simulink model "drone"  (R2020b)
settings: Solver=VariableStepAuto  StartTime=0.0  StopTime=3  RelTol=1e-3
values from neighbouring files (symbols this model uses):
  planta = obterPlanta()    [simularDrone.m]
  proj = obterProjeto()    [simularDrone.m]
libraries: pid_lib x6
settings Model: EnablePacing=on  Creator=kowalks  LastModifiedBy=kenji

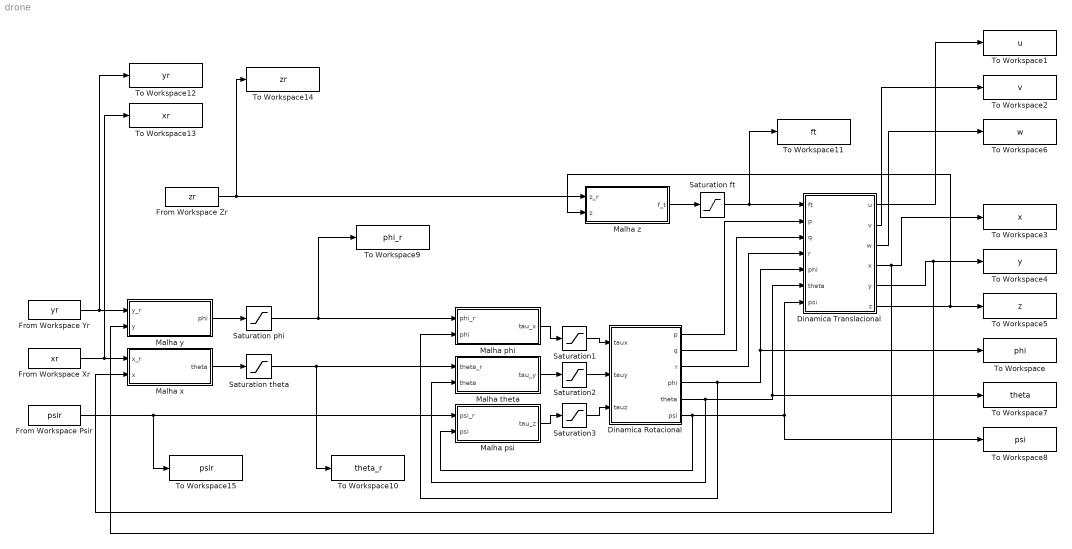
== system drone ==
  Dinamica Rotacional : Subsystem
  Dinamica Translacional : Subsystem
  From Workspace Psir : FromWorkspace  VariableName=psir
  From Workspace Xr : FromWorkspace  VariableName=xr
  From Workspace Yr : FromWorkspace  VariableName=yr
  From Workspace Zr : FromWorkspace  VariableName=zr
  Malha phi : Subsystem
  Malha psi : Subsystem
  Malha theta : Subsystem
  Malha x : Subsystem
  Malha y : Subsystem
  Malha z : Subsystem
  Saturation ft : Saturate  UpperLimit=2*planta.m*planta.g  LowerLimit=0.1*planta.m*planta.g
  Saturation phi : Saturate  UpperLimit=pi/6  LowerLimit=-pi/6
  Saturation theta : Saturate  UpperLimit=pi/6  LowerLimit=-pi/6
  Saturation1 : Saturate  UpperLimit=2*sqrt(2)*planta.l*planta.m*planta.g  LowerLimit=-2*sqrt(2)*planta.l*planta.m*planta.g
  Saturation2 : Saturate  UpperLimit=2*sqrt(2)*planta.l*planta.m*planta.g  LowerLimit=-2*sqrt(2)*planta.l*planta.m*planta.g
  Saturation3 : Saturate  UpperLimit=2*sqrt(2)*planta.l*planta.m*planta.g  LowerLimit=-2*sqrt(2)*planta.l*planta.m*planta.g
  To Workspace : ToWorkspace  VariableName=phi  SaveFormat=Timeseries  SampleTime=-1
  To Workspace1 : ToWorkspace  VariableName=u  SaveFormat=Timeseries  SampleTime=-1
  To Workspace10 : ToWorkspace  VariableName=theta_r  SaveFormat=Timeseries  SampleTime=-1
  To Workspace11 : ToWorkspace  VariableName=ft  SaveFormat=Timeseries  SampleTime=-1
  To Workspace12 : ToWorkspace  VariableName=yr  SaveFormat=Timeseries  SampleTime=-1
  To Workspace13 : ToWorkspace  VariableName=xr  SaveFormat=Timeseries  SampleTime=-1
  To Workspace14 : ToWorkspace  VariableName=zr  SaveFormat=Timeseries  SampleTime=-1
  To Workspace15 : ToWorkspace  VariableName=psir  SaveFormat=Timeseries  SampleTime=-1
  To Workspace2 : ToWorkspace  VariableName=v  SaveFormat=Timeseries  SampleTime=-1
  To Workspace3 : ToWorkspace  VariableName=x  SaveFormat=Timeseries  SampleTime=-1
  To Workspace4 : ToWorkspace  VariableName=y  SaveFormat=Timeseries  SampleTime=-1
  To Workspace5 : ToWorkspace  VariableName=z  SaveFormat=Timeseries  SampleTime=-1
  To Workspace6 : ToWorkspace  VariableName=w  SaveFormat=Timeseries  SampleTime=-1
  To Workspace7 : ToWorkspace  VariableName=theta  SaveFormat=Timeseries  SampleTime=-1
  To Workspace8 : ToWorkspace  VariableName=psi  SaveFormat=Timeseries  SampleTime=-1
  To Workspace9 : ToWorkspace  VariableName=phi_r  SaveFormat=Timeseries  SampleTime=-1
  wires:
  Dinamica Rotacional/6(psi) -> Malha psi/2(psi), Dinamica Translacional/7(psi), To Workspace8/1
  Dinamica Rotacional/5(theta) -> Malha theta/2(theta), To Workspace7/1, Dinamica Translacional/6(theta)
  Dinamica Rotacional/3(r) -> Dinamica Translacional/4(r)
  Dinamica Rotacional/2(q) -> Dinamica Translacional/3(q)
  Dinamica Rotacional/1(p) -> Dinamica Translacional/2(p)
  Dinamica Translacional/6(z) -> Malha z/2(z), To Workspace5/1
  Dinamica Translacional/5(y) -> Malha y/2(y), To Workspace4/1
  Dinamica Translacional/4(x) -> Malha x/2(x), To Workspace3/1
  Dinamica Translacional/3(w) -> To Workspace6/1
  Dinamica Translacional/2(v) -> To Workspace2/1
  Dinamica Translacional/1(u) -> To Workspace1/1
  From Workspace Xr/1 -> To Workspace13/1, Malha x/1(x_r)
  From Workspace Yr/1 -> To Workspace12/1, Malha y/1(y_r)
  From Workspace Psir/1 -> To Workspace15/1, Malha psi/1(psi_r)
  From Workspace Zr/1 -> To Workspace14/1, Malha z/1(z_r)
  Dinamica Rotacional/4(phi) -> Malha phi/2(phi), Dinamica Translacional/5(phi), To Workspace/1
  Malha y/1(phi) -> Saturation phi/1
  Malha x/1(theta) -> Saturation theta/1
  Saturation phi/1 -> To Workspace9/1, Malha phi/1(phi_r)
  Saturation theta/1 -> To Workspace10/1, Malha theta/1(theta_r)
  Malha z/1(f_t) -> Saturation ft/1
  Saturation ft/1 -> To Workspace11/1, Dinamica Translacional/1(ft)
  Malha phi/1(tau_x) -> Saturation1/1
  Saturation1/1 -> Dinamica Rotacional/1(taux)
  Saturation2/1 -> Dinamica Rotacional/2(tauy)
  Malha theta/1(tau_y) -> Saturation2/1
  Malha psi/1(tau_z) -> Saturation3/1
  Saturation3/1 -> Dinamica Rotacional/3(tauz)

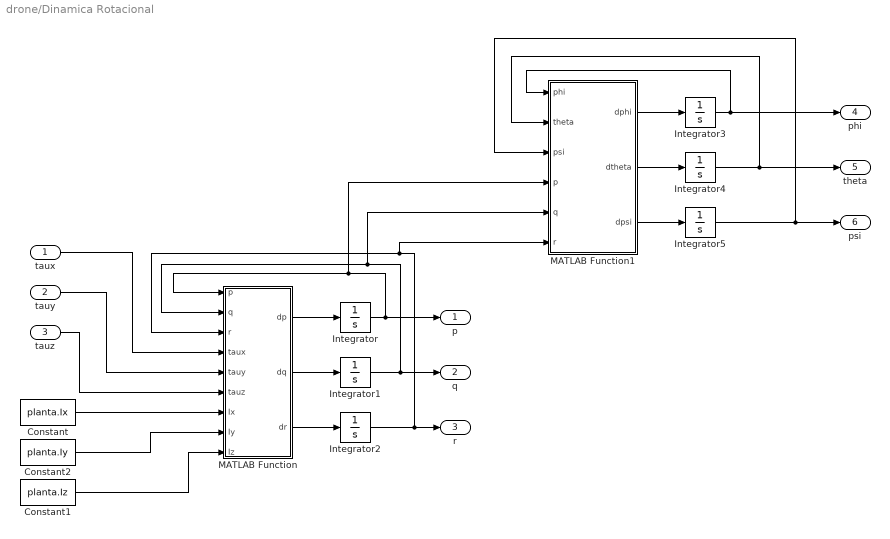
== system drone/Dinamica Rotacional ==
  taux : Inport
  tauy : Inport  Port=2
  tauz : Inport  Port=3
  Constant : Constant  Value=planta.Ix
  Constant1 : Constant  Value=planta.Iz
  Constant2 : Constant  Value=planta.Iy
  Integrator{,1..5} (6 alike) : Integrator
  MATLAB Function : MATLAB Function  TreatAsAtomicUnit=on
  MATLAB Function1 : MATLAB Function  TreatAsAtomicUnit=on
  p : Outport
  q : Outport  Port=2
  r : Outport  Port=3
  phi : Outport  Port=4
  theta : Outport  Port=5
  psi : Outport  Port=6
  wires:
  taux/1 -> MATLAB Function/4(taux)
  tauy/1 -> MATLAB Function/5(tauy)
  tauz/1 -> MATLAB Function/6(tauz)
  MATLAB Function/1(dp) -> Integrator/1
  MATLAB Function/2(dq) -> Integrator1/1
  MATLAB Function/3(dr) -> Integrator2/1
  Integrator1/1 -> q/1, MATLAB Function1/5(q), MATLAB Function/2(q)
  Integrator2/1 -> r/1, MATLAB Function1/6(r), MATLAB Function/3(r)
  Integrator/1 -> p/1, MATLAB Function1/4(p), MATLAB Function/1(p)
  Constant/1 -> MATLAB Function/7(Ix)
  Constant2/1 -> MATLAB Function/8(Iy)
  Constant1/1 -> MATLAB Function/9(Iz)
  MATLAB Function1/1(dphi) -> Integrator3/1
  MATLAB Function1/2(dtheta) -> Integrator4/1
  MATLAB Function1/3(dpsi) -> Integrator5/1
  Integrator3/1 -> MATLAB Function1/1(phi), phi/1
  Integrator4/1 -> theta/1, MATLAB Function1/2(theta)
  Integrator5/1 -> MATLAB Function1/3(psi), psi/1

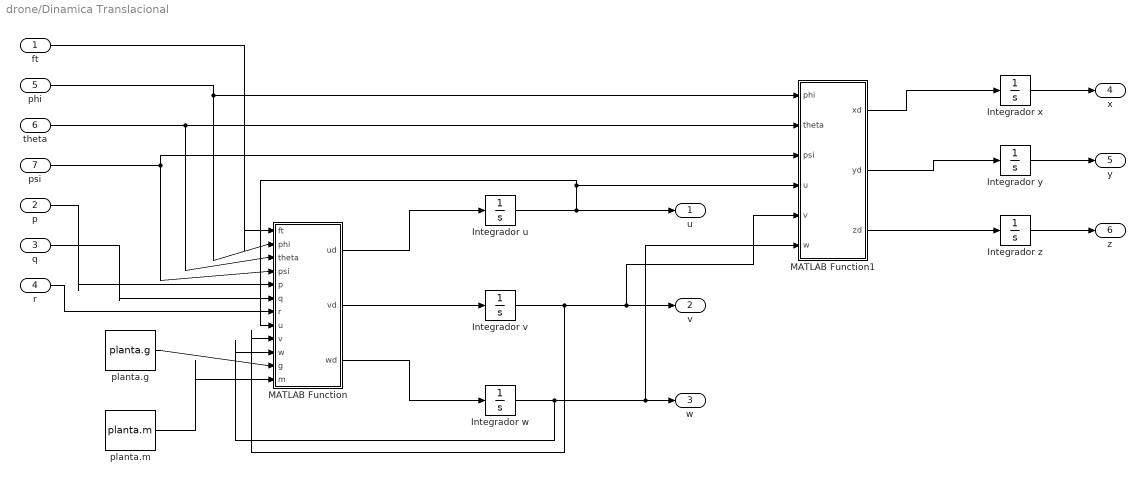
== system drone/Dinamica Translacional ==
  ft : Inport
  p : Inport  Port=2
  q : Inport  Port=3
  r : Inport  Port=4
  phi : Inport  Port=5
  theta : Inport  Port=6
  psi : Inport  Port=7
  Integrador u : Integrator
  Integrador v : Integrator
  Integrador w : Integrator
  Integrador x : Integrator
  Integrador y : Integrator
  Integrador z : Integrator
  MATLAB Function : MATLAB Function  TreatAsAtomicUnit=on
  MATLAB Function1 : MATLAB Function  TreatAsAtomicUnit=on
  planta.g : Constant  Value=planta.g
  planta.m : Constant  Value=planta.m
  u : Outport  PortDimensions=1
  v : Outport  Port=2  PortDimensions=1
  w : Outport  Port=3  PortDimensions=1
  x : Outport  Port=4  PortDimensions=1
  y : Outport  Port=5  PortDimensions=1
  z : Outport  Port=6  PortDimensions=1
  wires:
  phi/1 -> MATLAB Function/2(phi), MATLAB Function1/1(phi)
  theta/1 -> MATLAB Function/3(theta), MATLAB Function1/2(theta)
  psi/1 -> MATLAB Function/4(psi), MATLAB Function1/3(psi)
  ft/1 -> MATLAB Function/1(ft)
  MATLAB Function/1(ud) -> Integrador u/1
  MATLAB Function/2(vd) -> Integrador v/1
  MATLAB Function/3(wd) -> Integrador w/1
  Integrador w/1 -> MATLAB Function1/6(w), w/1, MATLAB Function/10(w)
  Integrador u/1 -> MATLAB Function/8(u), MATLAB Function1/4(u), u/1
  MATLAB Function1/2(yd) -> Integrador y/1
  MATLAB Function1/1(xd) -> Integrador x/1
  MATLAB Function1/3(zd) -> Integrador z/1
  p/1 -> MATLAB Function/5(p)
  q/1 -> MATLAB Function/6(q)
  r/1 -> MATLAB Function/7(r)
  Integrador v/1 -> MATLAB Function1/5(v), v/1, MATLAB Function/9(v)
  Integrador x/1 -> x/1
  Integrador y/1 -> y/1
  Integrador z/1 -> z/1
  planta.g/1 -> MATLAB Function/11(g)
  planta.m/1 -> MATLAB Function/12(m)

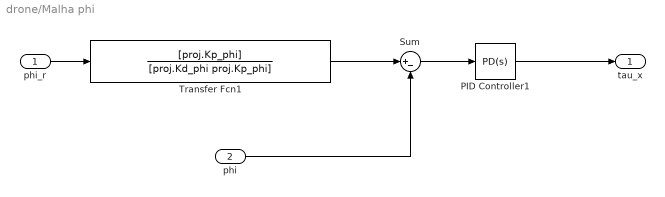
== system drone/Malha phi ==
  phi_r : Inport
  phi : Inport  Port=2
  PID Controller1 : pid_lib/PID Controller  Controller=PD  Form=Parallel  TimeDomain=Continuous-time  UseExternalTs=off  SampleTime=-1  IntegratorMethod=Forward Euler  FilterMethod=Forward Euler  ControllerParametersSource=internal  P=proj.Kp_phi  I=1  D=proj.Kd_phi  UseFilter=on  N=10000  TunerSelectOption=Transfer Function Based (PID Tuner App)  InitialConditionSource=internal  InitialConditionForIntegrator=0  InitialConditionForFilter=0  DifferentiatorICPrevScaledInput=0  ExternalReset=none  TrackingMode=off  Kt=1  LimitOutput=off  SatLimitsSource=internal  UpperSaturationLimit=inf  LowerSaturationLimit=-inf  LinearizeAsGain=on  AntiWindupMode=none  Kb=1  POutMin=[]  POutMax=[]  IOutMin=[]  IOutMax=[]  DOutMin=[]  DOutMax=[]  NOutMin=[]  NOutMax=[]  SumOutMin=[]  SumOutMax=[]  SaturationOutMin=[]  SaturationOutMax=[]  PParamMin=[]  PParamMax=[]  IParamMin=[]  IParamMax=[]  DParamMin=[]  DParamMax=[]  NParamMin=[]  NParamMax=[]  KbParamMin=[]  KbParamMax=[]  KtParamMin=[]  KtParamMax=[]  KbOutMin=[]  KbOutMax=[]  KtOutMin=[]  KtOutMax=[]  IntegratorOutMin=[]  IntegratorOutMax=[]  FilterOutMin=[]  FilterOutMax=[]  SumI1OutMin=[]  SumI1OutMax=[]  SumI2OutMin=[]  SumI2OutMax=[]  SumI3OutMin=[]  SumI3OutMax=[]  SumI4OutMin=[]  SumI4OutMax=[]  SumDOutMin=[]  SumDOutMax=[]  DifferentiatorOutMin=[]  DifferentiatorOutMax=[]  FilterDiffOutCoefMin=[]  FilterDiffOutCoefMax=[]  ReciprocalOutMin=[]  ReciprocalOutMax=[]  SumDenOutMin=[]  SumDenOutMax=[]  SumNumOutMin=[]  SumNumOutMax=[]  DivideOutMin=[]  DivideOutMax=[]  UdiffTsProdOutMin=[]  UdiffTsProdOutMax=[]  NTsProdOutMin=[]  NTsProdOutMax=[]  UintegralTsProdOutMin=[]  UintegralTsProdOutMax=[]  UngainTsProdOutMin=[]  UngainTsProdOutMax=[]  IntegratorContinuousStateAttributes=''  IntegratorStateMustResolveToSignalObject=off  IntegratorRTWStateStorageClass=Auto  FilterContinuousStateAttributes=''  FilterStateMustResolveToSignalObject=off  FilterRTWStateStorageClass=Auto  ParallelPVariant=InternalParameters  IdealPVariant=Disabled  IVariant=Disabled  DVariant=InternalParameters  IntegratorVariant=Disabled  SatVariant=Disabled  AWVariant=Disabled  PCopyVariant=Disabled  TRVariant=Disabled  FdbkBlocksVariant=Forward  IdealPFdbkVariant=Disabled  SatFdbkVariant=Disabled  DerivativeFilterVariant=ContFilter  NVariant=InternalParameters  NCopyVariant=Disabled  FilterICVariant=InternalICsFilter  IntegratorICVariant=Disabled  ExternalResetVariant=Disabled  TRSumVariant=Passthrough  SumFdbkVariant=Disabled  SumVariant=Sum_PD  TsampFilterVariant=InternalTs  TsampNgainVariant=Passthrough  TsampIntegralVariant=Disabled_SignalSpec  ExternalSaturationOutDataTypeStr=Inherit: Same as second input
  Sum : Sum  Inputs=|+-
  Transfer Fcn1 : TransferFcn  Numerator=[proj.Kp_phi]  Denominator=[proj.Kd_phi proj.Kp_phi]
  tau_x : Outport
  wires:
  phi_r/1 -> Transfer Fcn1/1
  Sum/1 -> PID Controller1/1
  Transfer Fcn1/1 -> Sum/1
  PID Controller1/1 -> tau_x/1
  phi/1 -> Sum/2

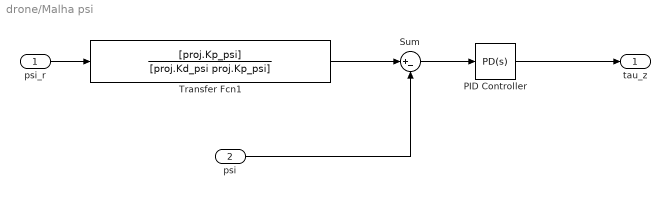
== system drone/Malha psi ==
  psi_r : Inport
  psi : Inport  Port=2
  PID Controller : pid_lib/PID Controller  Controller=PD  Form=Parallel  TimeDomain=Continuous-time  UseExternalTs=off  SampleTime=-1  IntegratorMethod=Forward Euler  FilterMethod=Forward Euler  ControllerParametersSource=internal  P=proj.Kp_psi  I=1  D=proj.Kd_psi  UseFilter=on  N=10000  TunerSelectOption=Transfer Function Based (PID Tuner App)  InitialConditionSource=internal  InitialConditionForIntegrator=0  InitialConditionForFilter=0  DifferentiatorICPrevScaledInput=0  ExternalReset=none  TrackingMode=off  Kt=1  LimitOutput=off  SatLimitsSource=internal  UpperSaturationLimit=inf  LowerSaturationLimit=-inf  LinearizeAsGain=on  AntiWindupMode=none  Kb=1  POutMin=[]  POutMax=[]  IOutMin=[]  IOutMax=[]  DOutMin=[]  DOutMax=[]  NOutMin=[]  NOutMax=[]  SumOutMin=[]  SumOutMax=[]  SaturationOutMin=[]  SaturationOutMax=[]  PParamMin=[]  PParamMax=[]  IParamMin=[]  IParamMax=[]  DParamMin=[]  DParamMax=[]  NParamMin=[]  NParamMax=[]  KbParamMin=[]  KbParamMax=[]  KtParamMin=[]  KtParamMax=[]  KbOutMin=[]  KbOutMax=[]  KtOutMin=[]  KtOutMax=[]  IntegratorOutMin=[]  IntegratorOutMax=[]  FilterOutMin=[]  FilterOutMax=[]  SumI1OutMin=[]  SumI1OutMax=[]  SumI2OutMin=[]  SumI2OutMax=[]  SumI3OutMin=[]  SumI3OutMax=[]  SumI4OutMin=[]  SumI4OutMax=[]  SumDOutMin=[]  SumDOutMax=[]  DifferentiatorOutMin=[]  DifferentiatorOutMax=[]  FilterDiffOutCoefMin=[]  FilterDiffOutCoefMax=[]  ReciprocalOutMin=[]  ReciprocalOutMax=[]  SumDenOutMin=[]  SumDenOutMax=[]  SumNumOutMin=[]  SumNumOutMax=[]  DivideOutMin=[]  DivideOutMax=[]  UdiffTsProdOutMin=[]  UdiffTsProdOutMax=[]  NTsProdOutMin=[]  NTsProdOutMax=[]  UintegralTsProdOutMin=[]  UintegralTsProdOutMax=[]  UngainTsProdOutMin=[]  UngainTsProdOutMax=[]  IntegratorContinuousStateAttributes=''  IntegratorStateMustResolveToSignalObject=off  IntegratorRTWStateStorageClass=Auto  FilterContinuousStateAttributes=''  FilterStateMustResolveToSignalObject=off  FilterRTWStateStorageClass=Auto  ParallelPVariant=InternalParameters  IdealPVariant=Disabled  IVariant=Disabled  DVariant=InternalParameters  IntegratorVariant=Disabled  SatVariant=Disabled  AWVariant=Disabled  PCopyVariant=Disabled  TRVariant=Disabled  FdbkBlocksVariant=Forward  IdealPFdbkVariant=Disabled  SatFdbkVariant=Disabled  DerivativeFilterVariant=ContFilter  NVariant=InternalParameters  NCopyVariant=Disabled  FilterICVariant=InternalICsFilter  IntegratorICVariant=Disabled  ExternalResetVariant=Disabled  TRSumVariant=Passthrough  SumFdbkVariant=Disabled  SumVariant=Sum_PD  TsampFilterVariant=InternalTs  TsampNgainVariant=Passthrough  TsampIntegralVariant=Disabled_SignalSpec  ExternalSaturationOutDataTypeStr=Inherit: Same as second input
  Sum : Sum  Inputs=|+-
  Transfer Fcn1 : TransferFcn  Numerator=[proj.Kp_psi]  Denominator=[proj.Kd_psi proj.Kp_psi]
  tau_z : Outport
  wires:
  psi/1 -> Sum/2
  PID Controller/1 -> tau_z/1
  psi_r/1 -> Transfer Fcn1/1
  Transfer Fcn1/1 -> Sum/1
  Sum/1 -> PID Controller/1

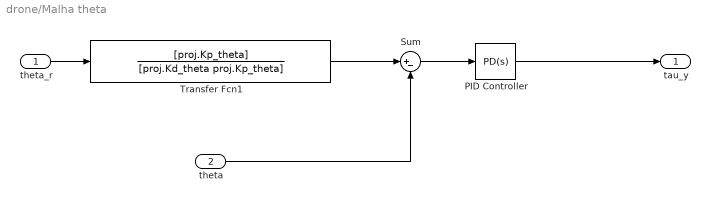
== system drone/Malha theta ==
  theta_r : Inport
  theta : Inport  Port=2
  PID Controller : pid_lib/PID Controller  Controller=PD  Form=Parallel  TimeDomain=Continuous-time  UseExternalTs=off  SampleTime=-1  IntegratorMethod=Forward Euler  FilterMethod=Forward Euler  ControllerParametersSource=internal  P=proj.Kp_theta  I=1  D=proj.Kd_theta  UseFilter=on  N=10000  TunerSelectOption=Transfer Function Based (PID Tuner App)  InitialConditionSource=internal  InitialConditionForIntegrator=0  InitialConditionForFilter=0  DifferentiatorICPrevScaledInput=0  ExternalReset=none  TrackingMode=off  Kt=1  LimitOutput=off  SatLimitsSource=internal  UpperSaturationLimit=planta.g*pi/6  LowerSaturationLimit=-planta.g*pi/6  LinearizeAsGain=off  AntiWindupMode=back-calculation  Kb=1  POutMin=[]  POutMax=[]  IOutMin=[]  IOutMax=[]  DOutMin=[]  DOutMax=[]  NOutMin=[]  NOutMax=[]  SumOutMin=[]  SumOutMax=[]  SaturationOutMin=[]  SaturationOutMax=[]  PParamMin=[]  PParamMax=[]  IParamMin=[]  IParamMax=[]  DParamMin=[]  DParamMax=[]  NParamMin=[]  NParamMax=[]  KbParamMin=[]  KbParamMax=[]  KtParamMin=[]  KtParamMax=[]  KbOutMin=[]  KbOutMax=[]  KtOutMin=[]  KtOutMax=[]  IntegratorOutMin=[]  IntegratorOutMax=[]  FilterOutMin=[]  FilterOutMax=[]  SumI1OutMin=[]  SumI1OutMax=[]  SumI2OutMin=[]  SumI2OutMax=[]  SumI3OutMin=[]  SumI3OutMax=[]  SumI4OutMin=[]  SumI4OutMax=[]  SumDOutMin=[]  SumDOutMax=[]  DifferentiatorOutMin=[]  DifferentiatorOutMax=[]  FilterDiffOutCoefMin=[]  FilterDiffOutCoefMax=[]  ReciprocalOutMin=[]  ReciprocalOutMax=[]  SumDenOutMin=[]  SumDenOutMax=[]  SumNumOutMin=[]  SumNumOutMax=[]  DivideOutMin=[]  DivideOutMax=[]  UdiffTsProdOutMin=[]  UdiffTsProdOutMax=[]  NTsProdOutMin=[]  NTsProdOutMax=[]  UintegralTsProdOutMin=[]  UintegralTsProdOutMax=[]  UngainTsProdOutMin=[]  UngainTsProdOutMax=[]  IntegratorContinuousStateAttributes=''  IntegratorStateMustResolveToSignalObject=off  IntegratorRTWStateStorageClass=Auto  FilterContinuousStateAttributes=''  FilterStateMustResolveToSignalObject=off  FilterRTWStateStorageClass=Auto  ParallelPVariant=InternalParameters  IdealPVariant=Disabled  IVariant=Disabled  DVariant=InternalParameters  IntegratorVariant=Disabled  SatVariant=Disabled  AWVariant=Disabled  PCopyVariant=Disabled  TRVariant=Disabled  FdbkBlocksVariant=Forward  IdealPFdbkVariant=Disabled  SatFdbkVariant=Disabled  DerivativeFilterVariant=ContFilter  NVariant=InternalParameters  NCopyVariant=Disabled  FilterICVariant=InternalICsFilter  IntegratorICVariant=Disabled  ExternalResetVariant=Disabled  TRSumVariant=Passthrough  SumFdbkVariant=Disabled  SumVariant=Sum_PD  TsampFilterVariant=InternalTs  TsampNgainVariant=Passthrough  TsampIntegralVariant=Disabled_SignalSpec  ExternalSaturationOutDataTypeStr=Inherit: Same as second input
  Sum : Sum  Inputs=|+-
  Transfer Fcn1 : TransferFcn  Numerator=[proj.Kp_theta]  Denominator=[proj.Kd_theta proj.Kp_theta]
  tau_y : Outport
  wires:
  theta_r/1 -> Transfer Fcn1/1
  Sum/1 -> PID Controller/1
  Transfer Fcn1/1 -> Sum/1
  theta/1 -> Sum/2
  PID Controller/1 -> tau_y/1

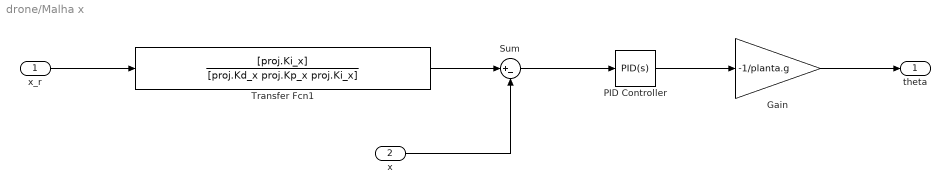
== system drone/Malha x ==
  x_r : Inport
  x : Inport  Port=2
  Gain : Gain  Gain=-1/planta.g
  PID Controller : pid_lib/PID Controller  Controller=PID  Form=Parallel  TimeDomain=Continuous-time  UseExternalTs=off  SampleTime=-1  IntegratorMethod=Forward Euler  FilterMethod=Forward Euler  ControllerParametersSource=internal  P=proj.Kp_x  I=proj.Ki_x  D=proj.Kd_x  UseFilter=on  N=10000000  TunerSelectOption=Transfer Function Based (PID Tuner App)  InitialConditionSource=internal  InitialConditionForIntegrator=0  InitialConditionForFilter=0  DifferentiatorICPrevScaledInput=0  ExternalReset=none  TrackingMode=off  Kt=1  LimitOutput=on  SatLimitsSource=internal  UpperSaturationLimit=planta.g*pi/6  LowerSaturationLimit=-planta.g*pi/6  LinearizeAsGain=off  AntiWindupMode=back-calculation  Kb=8  POutMin=[]  POutMax=[]  IOutMin=[]  IOutMax=[]  DOutMin=[]  DOutMax=[]  NOutMin=[]  NOutMax=[]  SumOutMin=[]  SumOutMax=[]  SaturationOutMin=[]  SaturationOutMax=[]  PParamMin=[]  PParamMax=[]  IParamMin=[]  IParamMax=[]  DParamMin=[]  DParamMax=[]  NParamMin=[]  NParamMax=[]  KbParamMin=[]  KbParamMax=[]  KtParamMin=[]  KtParamMax=[]  KbOutMin=[]  KbOutMax=[]  KtOutMin=[]  KtOutMax=[]  IntegratorOutMin=[]  IntegratorOutMax=[]  FilterOutMin=[]  FilterOutMax=[]  SumI1OutMin=[]  SumI1OutMax=[]  SumI2OutMin=[]  SumI2OutMax=[]  SumI3OutMin=[]  SumI3OutMax=[]  SumI4OutMin=[]  SumI4OutMax=[]  SumDOutMin=[]  SumDOutMax=[]  DifferentiatorOutMin=[]  DifferentiatorOutMax=[]  FilterDiffOutCoefMin=[]  FilterDiffOutCoefMax=[]  ReciprocalOutMin=[]  ReciprocalOutMax=[]  SumDenOutMin=[]  SumDenOutMax=[]  SumNumOutMin=[]  SumNumOutMax=[]  DivideOutMin=[]  DivideOutMax=[]  UdiffTsProdOutMin=[]  UdiffTsProdOutMax=[]  NTsProdOutMin=[]  NTsProdOutMax=[]  UintegralTsProdOutMin=[]  UintegralTsProdOutMax=[]  UngainTsProdOutMin=[]  UngainTsProdOutMax=[]  IntegratorContinuousStateAttributes=''  IntegratorStateMustResolveToSignalObject=off  IntegratorRTWStateStorageClass=Auto  FilterContinuousStateAttributes=''  FilterStateMustResolveToSignalObject=off  FilterRTWStateStorageClass=Auto  ParallelPVariant=InternalParameters  IdealPVariant=Disabled  IVariant=InternalParameters  DVariant=InternalParameters  IntegratorVariant=Continuous  SatVariant=Enabled  AWVariant=BackCalculation  PCopyVariant=Disabled  TRVariant=Disabled  FdbkBlocksVariant=Forward  IdealPFdbkVariant=Disabled  SatFdbkVariant=Disabled  DerivativeFilterVariant=ContFilter  NVariant=InternalParameters  NCopyVariant=Disabled  FilterICVariant=InternalICsFilter  IntegratorICVariant=InternalICs  ExternalResetVariant=Disabled  TRSumVariant=Passthrough  SumFdbkVariant=Disabled  SumVariant=Sum_PID  TsampFilterVariant=InternalTs  TsampNgainVariant=Passthrough  TsampIntegralVariant=Passthrough  ExternalSaturationOutDataTypeStr=Inherit: Same as second input
  Sum : Sum  Inputs=|+-
  Transfer Fcn1 : TransferFcn  Numerator=[proj.Ki_x]  Denominator=[proj.Kd_x proj.Kp_x proj.Ki_x]
  theta : Outport
  wires:
  Transfer Fcn1/1 -> Sum/1
  x/1 -> Sum/2
  x_r/1 -> Transfer Fcn1/1
  Sum/1 -> PID Controller/1
  PID Controller/1 -> Gain/1
  Gain/1 -> theta/1

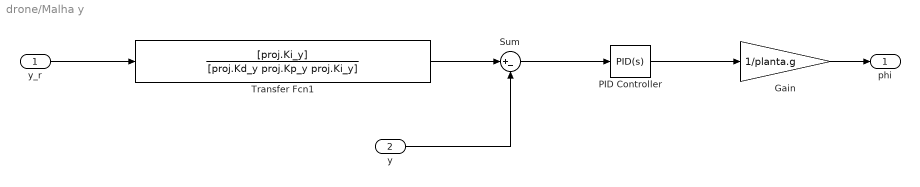
== system drone/Malha y ==
  y_r : Inport
  y : Inport  Port=2
  Gain : Gain  Gain=1/planta.g
  PID Controller : pid_lib/PID Controller  Controller=PID  Form=Parallel  TimeDomain=Continuous-time  UseExternalTs=off  SampleTime=-1  IntegratorMethod=Forward Euler  FilterMethod=Forward Euler  ControllerParametersSource=internal  P=proj.Kp_y  I=proj.Ki_y  D=proj.Kd_y  UseFilter=on  N=10000000  TunerSelectOption=Transfer Function Based (PID Tuner App)  InitialConditionSource=internal  InitialConditionForIntegrator=0  InitialConditionForFilter=0  DifferentiatorICPrevScaledInput=0  ExternalReset=none  TrackingMode=off  Kt=1  LimitOutput=on  SatLimitsSource=internal  UpperSaturationLimit=planta.g*pi/6  LowerSaturationLimit=-planta.g*pi/6  LinearizeAsGain=off  AntiWindupMode=back-calculation  Kb=8  POutMin=[]  POutMax=[]  IOutMin=[]  IOutMax=[]  DOutMin=[]  DOutMax=[]  NOutMin=[]  NOutMax=[]  SumOutMin=[]  SumOutMax=[]  SaturationOutMin=[]  SaturationOutMax=[]  PParamMin=[]  PParamMax=[]  IParamMin=[]  IParamMax=[]  DParamMin=[]  DParamMax=[]  NParamMin=[]  NParamMax=[]  KbParamMin=[]  KbParamMax=[]  KtParamMin=[]  KtParamMax=[]  KbOutMin=[]  KbOutMax=[]  KtOutMin=[]  KtOutMax=[]  IntegratorOutMin=[]  IntegratorOutMax=[]  FilterOutMin=[]  FilterOutMax=[]  SumI1OutMin=[]  SumI1OutMax=[]  SumI2OutMin=[]  SumI2OutMax=[]  SumI3OutMin=[]  SumI3OutMax=[]  SumI4OutMin=[]  SumI4OutMax=[]  SumDOutMin=[]  SumDOutMax=[]  DifferentiatorOutMin=[]  DifferentiatorOutMax=[]  FilterDiffOutCoefMin=[]  FilterDiffOutCoefMax=[]  ReciprocalOutMin=[]  ReciprocalOutMax=[]  SumDenOutMin=[]  SumDenOutMax=[]  SumNumOutMin=[]  SumNumOutMax=[]  DivideOutMin=[]  DivideOutMax=[]  UdiffTsProdOutMin=[]  UdiffTsProdOutMax=[]  NTsProdOutMin=[]  NTsProdOutMax=[]  UintegralTsProdOutMin=[]  UintegralTsProdOutMax=[]  UngainTsProdOutMin=[]  UngainTsProdOutMax=[]  IntegratorContinuousStateAttributes=''  IntegratorStateMustResolveToSignalObject=off  IntegratorRTWStateStorageClass=Auto  FilterContinuousStateAttributes=''  FilterStateMustResolveToSignalObject=off  FilterRTWStateStorageClass=Auto  ParallelPVariant=InternalParameters  IdealPVariant=Disabled  IVariant=InternalParameters  DVariant=InternalParameters  IntegratorVariant=Continuous  SatVariant=Enabled  AWVariant=BackCalculation  PCopyVariant=Disabled  TRVariant=Disabled  FdbkBlocksVariant=Forward  IdealPFdbkVariant=Disabled  SatFdbkVariant=Disabled  DerivativeFilterVariant=ContFilter  NVariant=InternalParameters  NCopyVariant=Disabled  FilterICVariant=InternalICsFilter  IntegratorICVariant=InternalICs  ExternalResetVariant=Disabled  TRSumVariant=Passthrough  SumFdbkVariant=Disabled  SumVariant=Sum_PID  TsampFilterVariant=InternalTs  TsampNgainVariant=Passthrough  TsampIntegralVariant=Passthrough  ExternalSaturationOutDataTypeStr=Inherit: Same as second input
  Sum : Sum  Inputs=|+-
  Transfer Fcn1 : TransferFcn  Numerator=[proj.Ki_y]  Denominator=[proj.Kd_y proj.Kp_y proj.Ki_y]
  phi : Outport
  wires:
  y/1 -> Sum/2
  y_r/1 -> Transfer Fcn1/1
  Transfer Fcn1/1 -> Sum/1
  Gain/1 -> phi/1
  Sum/1 -> PID Controller/1
  PID Controller/1 -> Gain/1

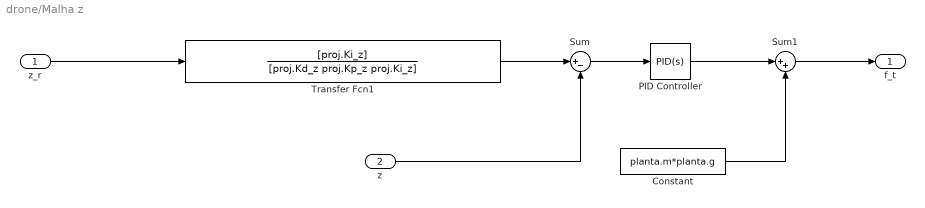
== system drone/Malha z ==
  z_r : Inport
  z : Inport  Port=2
  Constant : Constant  Value=planta.m*planta.g
  PID Controller : pid_lib/PID Controller  Controller=PID  Form=Parallel  TimeDomain=Continuous-time  UseExternalTs=off  SampleTime=-1  IntegratorMethod=Forward Euler  FilterMethod=Forward Euler  ControllerParametersSource=internal  P=proj.Kp_z  I=proj.Ki_z  D=proj.Kd_z  UseFilter=on  N=10000000  TunerSelectOption=Transfer Function Based (PID Tuner App)  InitialConditionSource=internal  InitialConditionForIntegrator=0  InitialConditionForFilter=0  DifferentiatorICPrevScaledInput=0  ExternalReset=none  TrackingMode=off  Kt=1  LimitOutput=on  SatLimitsSource=internal  UpperSaturationLimit=planta.m*planta.g  LowerSaturationLimit=-planta.m*planta.g  LinearizeAsGain=on  AntiWindupMode=back-calculation  Kb=8  POutMin=[]  POutMax=[]  IOutMin=[]  IOutMax=[]  DOutMin=[]  DOutMax=[]  NOutMin=[]  NOutMax=[]  SumOutMin=[]  SumOutMax=[]  SaturationOutMin=[]  SaturationOutMax=[]  PParamMin=[]  PParamMax=[]  IParamMin=[]  IParamMax=[]  DParamMin=[]  DParamMax=[]  NParamMin=[]  NParamMax=[]  KbParamMin=[]  KbParamMax=[]  KtParamMin=[]  KtParamMax=[]  KbOutMin=[]  KbOutMax=[]  KtOutMin=[]  KtOutMax=[]  IntegratorOutMin=[]  IntegratorOutMax=[]  FilterOutMin=[]  FilterOutMax=[]  SumI1OutMin=[]  SumI1OutMax=[]  SumI2OutMin=[]  SumI2OutMax=[]  SumI3OutMin=[]  SumI3OutMax=[]  SumI4OutMin=[]  SumI4OutMax=[]  SumDOutMin=[]  SumDOutMax=[]  DifferentiatorOutMin=[]  DifferentiatorOutMax=[]  FilterDiffOutCoefMin=[]  FilterDiffOutCoefMax=[]  ReciprocalOutMin=[]  ReciprocalOutMax=[]  SumDenOutMin=[]  SumDenOutMax=[]  SumNumOutMin=[]  SumNumOutMax=[]  DivideOutMin=[]  DivideOutMax=[]  UdiffTsProdOutMin=[]  UdiffTsProdOutMax=[]  NTsProdOutMin=[]  NTsProdOutMax=[]  UintegralTsProdOutMin=[]  UintegralTsProdOutMax=[]  UngainTsProdOutMin=[]  UngainTsProdOutMax=[]  IntegratorContinuousStateAttributes=''  IntegratorStateMustResolveToSignalObject=off  IntegratorRTWStateStorageClass=Auto  FilterContinuousStateAttributes=''  FilterStateMustResolveToSignalObject=off  FilterRTWStateStorageClass=Auto  ParallelPVariant=InternalParameters  IdealPVariant=Disabled  IVariant=InternalParameters  DVariant=InternalParameters  IntegratorVariant=Continuous  SatVariant=Enabled  AWVariant=BackCalculation  PCopyVariant=Disabled  TRVariant=Disabled  FdbkBlocksVariant=Forward  IdealPFdbkVariant=Disabled  SatFdbkVariant=Disabled  DerivativeFilterVariant=ContFilter  NVariant=InternalParameters  NCopyVariant=Disabled  FilterICVariant=InternalICsFilter  IntegratorICVariant=InternalICs  ExternalResetVariant=Disabled  TRSumVariant=Passthrough  SumFdbkVariant=Disabled  SumVariant=Sum_PID  TsampFilterVariant=InternalTs  TsampNgainVariant=Passthrough  TsampIntegralVariant=Passthrough  ExternalSaturationOutDataTypeStr=Inherit: Same as second input
  Sum : Sum  Inputs=|+-
  Sum1 : Sum  Inputs=|++
  Transfer Fcn1 : TransferFcn  Numerator=[proj.Ki_z]  Denominator=[proj.Kd_z proj.Kp_z proj.Ki_z]
  f_t : Outport
  wires:
  Transfer Fcn1/1 -> Sum/1
  Sum/1 -> PID Controller/1
  z_r/1 -> Transfer Fcn1/1
  z/1 -> Sum/2
  PID Controller/1 -> Sum1/1
  Sum1/1 -> f_t/1
  Constant/1 -> Sum1/2

== matlab function drone/Dinamica Translacional/MATLAB Function1 ==
  data: phi input; theta input; psi input; u input; xd output; v input; w input; yd output; zd output
function [xd, yd, zd] = fcn(phi, theta, psi, u, v, w)

    xd1 = cos(psi)*cos(theta)*u;
    xd2 = (cos(psi)*sin(phi)*sin(theta)-cos(phi)*sin(psi))*v;
    xd3 = (sin(phi)*sin(psi)+cos(phi)*cos(psi)*sin(theta))*w;
    xd = xd1+xd2+xd3;
    
    yd1 = cos(theta)*sin(psi)*u;
    yd2 = (cos(phi)*cos(psi)+sin(phi)*sin(psi)*sin(theta))*v;
    yd3 = (cos(phi)*sin(psi)*sin(theta)-cos(psi)*sin(phi))*w;
    yd = yd1+yd2+yd3;
    
    zd = -sin(theta)*u + cos(theta)*sin(phi)*v + cos(phi)*cos(theta)*w;
    
end

== matlab function drone/Dinamica Translacional/MATLAB Function ==
  data: ft input; phi input; theta input; psi input; p input; q input; r input; u input; ud output; v input; w input; vd output; wd output; g input; m input
function [ud, vd, wd] = fcn(ft,  phi, theta, psi, p, q, r, u, v, w, g,m)

    ud = r*v - q*w - g * sin(theta);
    vd = -r*u + p*w + g * sin(phi)*cos(theta);
    wd = q*u - p*v + g * cos(phi)*cos(theta) - ft/m;

end

== matlab function drone/Dinamica Rotacional/MATLAB Function ==
  data: p input; q input; r input; taux input; dp output; tauy input; tauz input; Ix input; Iy input; Iz input; dq output; dr output
function [dp, dq, dr]= fcn(p, q, r, taux, tauy, tauz, Ix, Iy, Iz)
    dp = (Iy-Iz)/Ix*r*q + taux/Ix;
    dq = (Iz-Ix)/Iy*p*r + tauy/Iy;
    dr = (Ix-Iy)/Iz*p*q + tauz/Iz;
end

== matlab function drone/Dinamica Rotacional/MATLAB Function1 ==
  data: phi input; dphi output; theta input; psi input; p input; q input; r input; dtheta output; dpsi output
function [dphi, dtheta, dpsi]= fcn(phi, theta, psi, p, q, r)
    dphi = p + sin(phi)*tan(theta)*q + cos(phi)*tan(theta)*r;
    dtheta = q*cos(phi) - r*sin(phi);
    dpsi = (q*sin(phi) + r*cos(phi))/cos(theta);

end
